simulink model "Simul3"  (R2019b)
settings: Solver=ode4  StartTime=0.0  StopTime=2  FixedStep=0.0005  RelTol=1e-3
values from neighbouring files (symbols this model uses):
  D = 0.003    [parameter.m]
  den_a = [1 2*zeta*omega_a(2) omega_a(2)^2]    [parameter.m]
  den_s = [1 2*zeta*omega_s omega_s^2]    [parameter.m]
  Ldelta = 16000    [parameter.m]
  Lp = 3.2    [parameter.m]
  Lpi = 1200    [parameter.m]
  num_a = [omega_a(2)^2]    [parameter.m]
  num_s = [omega_s^2]    [parameter.m]
  P = [0.94 0.96 1.00 1.05 1.07 1.09 1.14 1.17 1.21 1.24 1.28]    [HW3_1.m]    (also in parameter.m = 27)
  theta_c = [pi/4 pi/8 0]    [parameter.m]
settings Model: Creator=MoonSunBeen  LastModifiedBy=MoonSunBeen

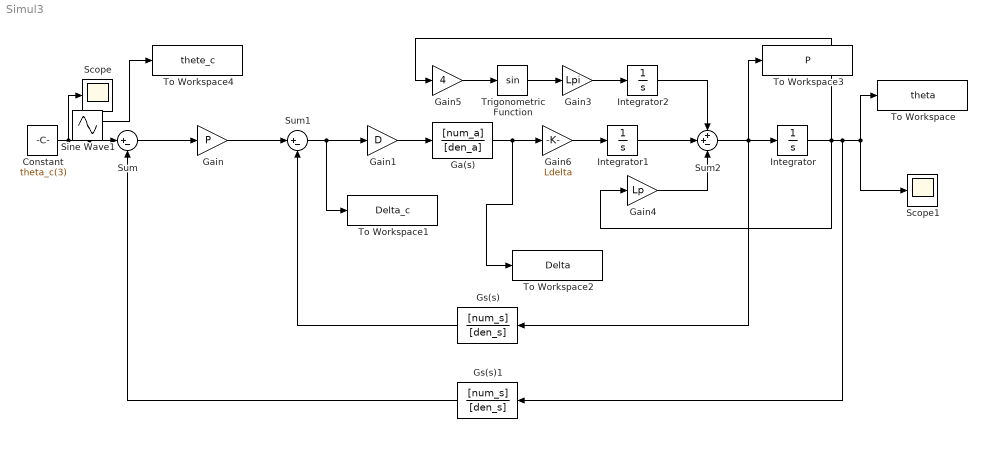
== system Simul3 ==
  Constant : Constant  Value=theta_c(3)
  Ga(s) : TransferFcn  Numerator=[num_a]  Denominator=[den_a]
  Gain : Gain  Gain=P
  Gain1 : Gain  Gain=D
  Gain3 : Gain  Gain=Lpi
  Gain4 : Gain  Gain=Lp
  Gain5 : Gain  Gain=4
  Gain6 : Gain  Gain=Ldelta
  Gs(s) : TransferFcn  Numerator=[num_s]  Denominator=[den_s]
  Gs(s)1 : TransferFcn  Numerator=[num_s]  Denominator=[den_s]
  Integrator : Integrator
  Integrator1 : Integrator
  Integrator2 : Integrator
  Scope : Scope
  Scope1 : Scope
  Sum : Sum  Inputs=|+-
  Sum1 : Sum  Inputs=|+-
  Sum2 : Sum  Inputs=++-
  To Workspace : ToWorkspace  VariableName=theta  SampleTime=-1
  To Workspace1 : ToWorkspace  VariableName=Delta_c  SampleTime=-1
  To Workspace2 : ToWorkspace  VariableName=Delta  SampleTime=-1
  To Workspace3 : ToWorkspace  VariableName=P  SampleTime=-1
  To Workspace4 : ToWorkspace  VariableName=thete_c  SampleTime=-1
  Trigonometric Function : Trigonometry
  Sine Wave1 : Sin  IOType=siggen  SampleTime=0
  wires:
  Sum/1 -> Gain/1
  Gain/1 -> Sum1/1
  Sum1/1 -> To Workspace1/1, Gain1/1
  Gain1/1 -> Ga(s)/1
  Gs(s)/1 -> Sum1/2
  Gs(s)1/1 -> Sum/2
  Constant/1 -> Scope/1, To Workspace4/1, Sum/1
  Sum2/1 -> To Workspace3/1, Integrator/1, Gs(s)/1
  Trigonometric Function/1 -> Gain3/1
  Gain5/1 -> Trigonometric Function/1
  Ga(s)/1 -> To Workspace2/1, Gain6/1
  Gain6/1 -> Integrator1/1
  Integrator1/1 -> Sum2/2
  Gain4/1 -> Sum2/3
  Integrator2/1 -> Sum2/1
  Gain3/1 -> Integrator2/1
  Integrator/1 -> Gain4/1, Gain5/1, Gs(s)1/1, Scope1/1, To Workspace/1
